simulink model "sim_orbit_min"  (Simulink 10.3)
settings: Solver=VariableStepAuto  StartTime=0.0  StopTime=.05*24*3600  FixedStep=1  MaxStep=1  RelTol=1e-3
InitFcn:
  | INIT_parametros;
  | dataAtm = data_atm('US1976');
undefined symbols (not defined in the file): A_transversal, a_world, b_world, Cbar, CI_angular, CI_lineal, e2_world, es2_world, GM, GRAV_MODEL, I, Jw, K, L, m, Omega0, Omega_max, P_peak, r_CG_in_G, SAT_SHAPE, Sbar, solar_cosep, solar_sinep, u_peak, WMM2025
libraries: aerolibgravity2 x1
settings Model: Creator=Allan  LastModifiedBy=RUSSO.MARTINEZ
settings SolverCC: AlgebraicLoopSolver=Auto
settings DataIOCC: SaveFormat=Dataset  SignalLoggingSaveFormat=Dataset
settings OptimizationCC: BlockReduction=off  ExpressionDepthLimit=128  LifeSpan=auto
settings DebuggingCC: SignalInfNanChecking=error  AlgebraicLoopMsg=none  UnderspecifiedInitializationDetection=Simplified  MergeDetectMultiDrivingBlocksExec=error  FcnCallInpInsideContextMsg=error  UnconnectedInputMsg=none  UnconnectedOutputMsg=none  UnconnectedLineMsg=none  StateNameClashWarn=none  SFUnexpectedBacktrackingDiag=error  SFNoUnconditionalDefaultTransitionDiag=error  SFExecutionAtInitializationDiag=warning  ArithmeticOperatorsInVariantConditions=error
settings HardwareCC: ProdBitPerPointer=64  ProdBitPerSizeT=64  ProdBitPerPtrDiffT=64  ProdLargestAtomicFloat=Float  ProdIntDivRoundTo=Zero  ProdEndianess=LittleEndian  ProdWordSize=64  ProdHWDeviceType=Intel->x86-64 (Windows64)
settings ModelReferenceCC: EnableRefExpFcnMdlSchedulingChecks=off  PropagateSignalLabelsOutOfModel=on
settings SFSimCC: SimUseLocalCustomCode=on  CustomCodeUndefinedFunction=FilterOut
settings RTWCC: RTWUseLocalCustomCode=on  GPUComputeCapability=5.0  DLArmComputeVersion=20.02.1
settings CodeAppCC: StateflowObjectComments=off
settings GRTTargetCC: TargetLangStandard=C99 (ISO)  CombineOutputUpdateFcns=on  GRTInterface=off
settings ConfigComp: CovMetricSettings=dwe  CovSaveCumulativeToWorkspaceVar=off  CovSaveSingleToWorkspaceVar=off  CovExternalEMLEnable=on  CovBoundaryAbsTol=1.0e-5

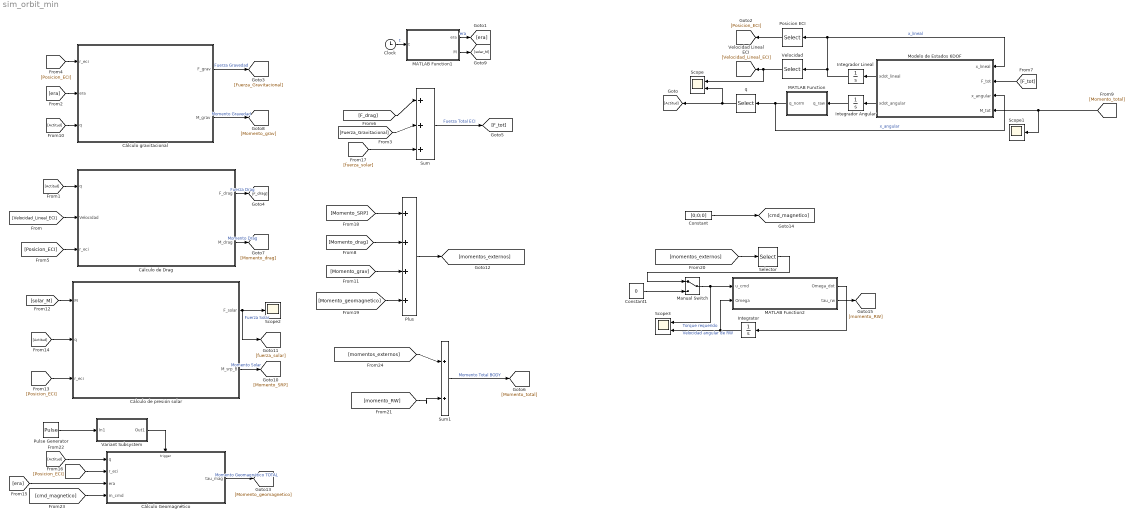
== system sim_orbit_min ==
  Clock : Clock
  Constant : Constant  Value=[0;0;0]  VectorParams1D=off
  Constant1 : Constant  Value=0
  Cálculo Geomagnético : Subsystem
  Cálculo de Drag : Subsystem
  Cálculo de presión solar : Subsystem
  Cálculo gravitacional : Subsystem
  Integrador Angular : Integrator  InitialCondition=CI_angular
  Integrador Lineal : Integrator  InitialCondition=CI_lineal
  Integrator : Integrator  InitialCondition=Omega0
  MATLAB Function : MATLAB Function  TreatAsAtomicUnit=on
  MATLAB Function1 : MATLAB Function  Priority=2  TreatAsAtomicUnit=on
  MATLAB Function2 : MATLAB Function  TreatAsAtomicUnit=on
  Manual Switch : ManualSwitch
  Modelo de Estados 6DOF : MATLAB Function  TreatAsAtomicUnit=on
  Plus : Sum  Inputs=++++
  Posicion ECI : Selector  InputPortWidth=6  IndexOptions=Index vector (dialog)  Indices=[1 2 3]  OutputSizes=1
  Pulse Generator : DiscretePulseGenerator  PulseType=Time based  Period=1  PulseWidth=50
  Scope : Scope  NumInputPorts=2
  Scope1 : Scope
  Scope2 : Scope
  Scope3 : Scope  NumInputPorts=2
  Selector : Selector  InputPortWidth=3  IndexOptions=Index vector (dialog)  Indices=[1]  OutputSizes=1
  Sum : Sum  Inputs=|+++
  Sum1 : Sum  Inputs=+|+
  Variant Subsystem : Subsystem  Variant=on
  "Velocidad " : Selector  InputPortWidth=6  IndexOptions=Index vector (dialog)  Indices=[4 5 6]  OutputSizes=1
  q : Selector  InputPortWidth=7  IndexOptions=Index vector (dialog)  Indices=[1 2 3 4]  OutputSizes=1
  wires:
  Clock/1 -> MATLAB Function1/1(t)  "t"
  Integrador Lineal/1 -> Posicion ECI/1, Modelo de Estados 6DOF/1(x_lineal), "Velocidad "/1  "x_lineal"
  "Velocidad "/1 -> Scope/1, [Velocidad_Lineal_ECI]
  Modelo de Estados 6DOF/1(xdot_lineal) -> Integrador Lineal/1
  Integrador Angular/1 -> MATLAB Function/1(q_raw)
  [Momento_total] -> Scope1/1, Modelo de Estados 6DOF/4(M_tot)
  [Actitud] -> Cálculo de Drag/1(q)
  [Velocidad_Lineal_ECI] -> Cálculo de Drag/2(Velocidad)
  MATLAB Function1/1(era) -> [era]  "era"
  Posicion ECI/1 -> [Posicion_ECI]
  [Posicion_ECI] -> Cálculo de Drag/3(r_eci)
  [era] -> Cálculo gravitacional/2(era)
  [Posicion_ECI] -> Cálculo gravitacional/1(r_eci)
  Cálculo gravitacional/1(F_grav) -> [Fuerza_Gravitacional]  "Fuerza Gravedad"
  [F_tot] -> Modelo de Estados 6DOF/2(F_tot)
  Modelo de Estados 6DOF/2(xdot_angular) -> Integrador Angular/1
  Cálculo de Drag/1(F_drag) -> [F_drag]  "Fuerza Drag"
  [F_drag] -> Sum/1
  Sum/1 -> [F_tot]  "Fuerza Total ECI"
  [Fuerza_Gravitacional] -> Sum/2
  Sum1/1 -> [Momento_total]  "Momento Total BODY"
  Cálculo de Drag/2(M_drag) -> [Momento_drag]  "Momento Drag"
  [Actitud] -> Cálculo gravitacional/3(q)
  Cálculo gravitacional/2(M_grav) -> [Momento_grav]  "Momento Gravedad"
  MATLAB Function1/2(M) -> [solar_M]
  [fuerza_solar] -> Sum/3
  [solar_M] -> Cálculo de presión solar/1(M)
  [Actitud] -> Cálculo de presión solar/2(q)
  [Posicion_ECI] -> Cálculo de presión solar/3(r_eci)
  Cálculo de presión solar/1(F_solar) -> [fuerza_solar], Scope2/1  "Fuerza Solar"
  Constant/1 -> [cmd_magnetico]
  [Actitud] -> Cálculo Geomagnético/1(q)
  [Posicion_ECI] -> Cálculo Geomagnético/2(r_eci)
  [era] -> Cálculo Geomagnético/3(era)
  [cmd_magnetico] -> Cálculo Geomagnético/4(m_cmd)
  Cálculo Geomagnético/1(tau_mag) -> [Momento_geomagnetico]  "Momento Geomagnético TOTAL"
  q/1 -> Scope/2, [Actitud]
  MATLAB Function/1(q_norm) -> Modelo de Estados 6DOF/3(x_angular), q/1  "x_angular"
  Cálculo de presión solar/2(M_srp_B) -> [Momento_SRP]  "Momento Solar"
  Pulse Generator/1 -> Variant Subsystem/1(In1)
  Variant Subsystem/1(Out1) -> Cálculo Geomagnético/Trigger
  [Momento_geomagnetico] -> Plus/4
  [Momento_grav] -> Plus/3
  [Momento_drag] -> Plus/2
  [Momento_SRP] -> Plus/1
  Plus/1 -> [momentos_externos]
  MATLAB Function2/1(Omega_dot) -> Integrator/1
  Integrator/1 -> MATLAB Function2/2(Omega), Scope3/2  "Velocidad angular de RW"
  [momentos_externos] -> Selector/1
  MATLAB Function2/2(tau_rw) -> [momento_RW]
  [momento_RW] -> Sum1/2
  [momentos_externos] -> Sum1/1
  Manual Switch/1 -> Scope3/1, MATLAB Function2/1(u_cmd)  "Torque requerido"
  Selector/1 -> Manual Switch/1
  Constant1/1 -> Manual Switch/2

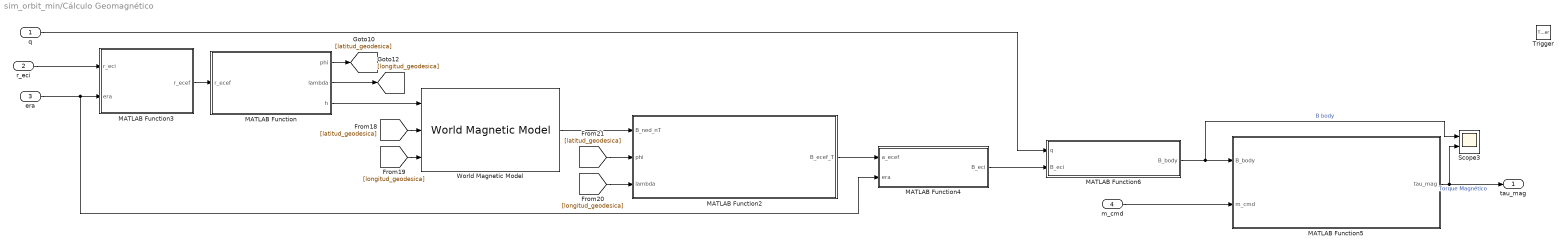
== system sim_orbit_min/Cálculo Geomagnético ==
  q : Inport
  r_eci : Inport  Port=2
  era : Inport  Port=3
  m_cmd : Inport  Port=4
  Trigger : TriggerPort  VariantControl=(inherit)  PortDimensions=1
  MATLAB Function : MATLAB Function  TreatAsAtomicUnit=on
  MATLAB Function2 : MATLAB Function  TreatAsAtomicUnit=on
  MATLAB Function3 : MATLAB Function  Priority=4  TreatAsAtomicUnit=on
  MATLAB Function4 : MATLAB Function  TreatAsAtomicUnit=on
  MATLAB Function5 : MATLAB Function  TreatAsAtomicUnit=on
  MATLAB Function6 : MATLAB Function  TreatAsAtomicUnit=on
  Scope3 : Scope  NumInputPorts=2
  World Magnetic Model : aerolibgravity2/World Magnetic Model  model=WMM2025 (2025-2030)  customFile='WMM2025.COF'  units=Metric (MKS)  time_in=off  month=January  day=1  year=2025  action=Error  h_out=off  dec_out=off  inc_out=off  ti_out=off
  tau_mag : Outport
  wires:
  [latitud_geodesica] -> MATLAB Function2/2(phi)
  [longitud_geodesica] -> World Magnetic Model/3
  MATLAB Function5/1(tau_mag) -> tau_mag/1, Scope3/2  "Torque Magnético"
  m_cmd/1 -> MATLAB Function5/2(m_cmd)
  MATLAB Function/1(phi) -> [latitud_geodesica]
  [latitud_geodesica] -> World Magnetic Model/2
  era/1 -> MATLAB Function4/2(era), MATLAB Function3/2(era)
  MATLAB Function6/1(B_body) -> Scope3/1, MATLAB Function5/1(B_body)  "B body"
  MATLAB Function/3(h) -> World Magnetic Model/1
  q/1 -> MATLAB Function6/1(q)
  [longitud_geodesica] -> MATLAB Function2/3(lambda)
  MATLAB Function/2(lambda) -> [longitud_geodesica]
  MATLAB Function4/1(B_eci) -> MATLAB Function6/2(B_eci)
  MATLAB Function2/1(B_ecef_T) -> MATLAB Function4/1(a_ecef)
  MATLAB Function3/1(r_ecef) -> MATLAB Function/1(r_ecef)
  World Magnetic Model/1 -> MATLAB Function2/1(B_ned_nT)
  r_eci/1 -> MATLAB Function3/1(r_eci)

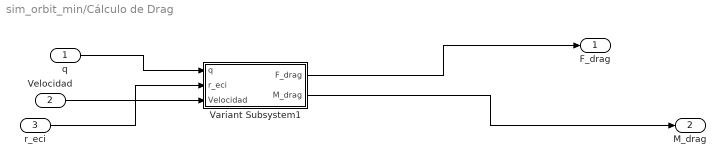
== system sim_orbit_min/Cálculo de Drag ==
  q : Inport
  Velocidad : Inport  Port=2
  r_eci : Inport  Port=3
  Variant Subsystem1 : Subsystem  Variant=on
  F_drag : Outport
  M_drag : Outport  Port=2  VectorParamsAs1DForOutWhenUnconnected=off
  wires:
  q/1 -> Variant Subsystem1/1(q)
  Velocidad/1 -> Variant Subsystem1/3(Velocidad)
  r_eci/1 -> Variant Subsystem1/2(r_eci)
  Variant Subsystem1/1(F_drag) -> F_drag/1
  Variant Subsystem1/2(M_drag) -> M_drag/1

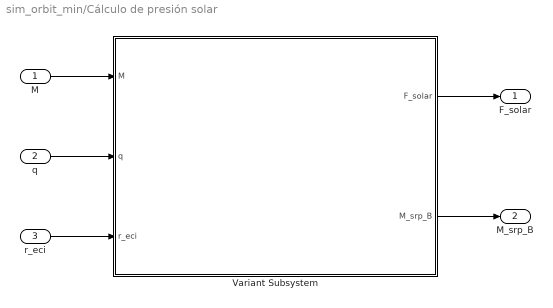
== system sim_orbit_min/Cálculo de presión solar ==
  M : Inport
  q : Inport  Port=2
  r_eci : Inport  Port=3
  Variant Subsystem : Subsystem  Variant=on
  F_solar : Outport
  M_srp_B : Outport  Port=2  VectorParamsAs1DForOutWhenUnconnected=off
  wires:
  M/1 -> Variant Subsystem/1(M)
  r_eci/1 -> Variant Subsystem/3(r_eci)
  q/1 -> Variant Subsystem/2(q)
  Variant Subsystem/1(F_solar) -> F_solar/1
  Variant Subsystem/2(M_srp_B) -> M_srp_B/1

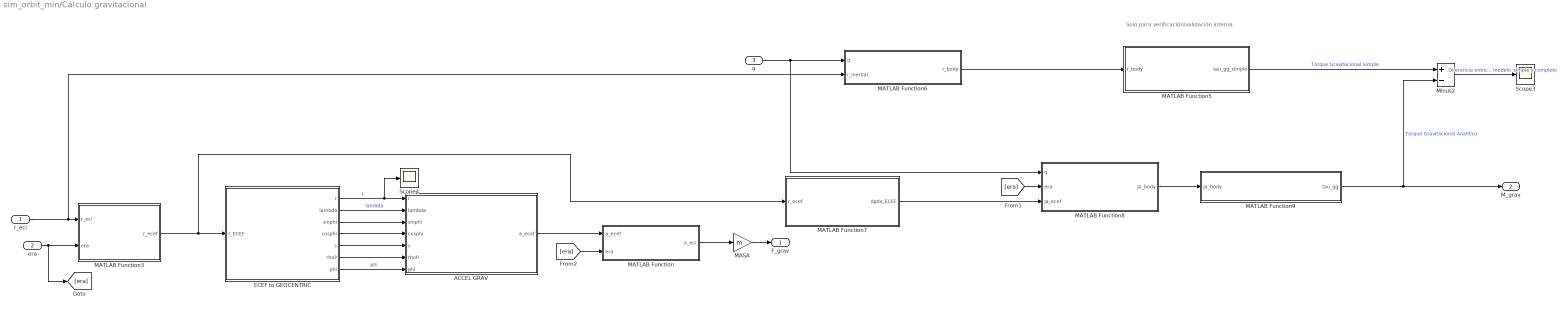
== system sim_orbit_min/Cálculo gravitacional ==
  note: Solo para verificación/validación interna.
  r_eci : Inport
  era : Inport  Port=2
  q : Inport  Port=3
  ACCEL GRAV : MATLAB Function  TreatAsAtomicUnit=on
  ECEF to GEOCENTRIC : MATLAB Function  TreatAsAtomicUnit=on
  MASA : Gain  Gain=m
  MATLAB Function : MATLAB Function  TreatAsAtomicUnit=on
  MATLAB Function3 : MATLAB Function  Priority=4  TreatAsAtomicUnit=on
  MATLAB Function5 : MATLAB Function  TreatAsAtomicUnit=on
  MATLAB Function6 : MATLAB Function  TreatAsAtomicUnit=on
  MATLAB Function7 : MATLAB Function  TreatAsAtomicUnit=on
  MATLAB Function8 : MATLAB Function  TreatAsAtomicUnit=on
  MATLAB Function9 : MATLAB Function  TreatAsAtomicUnit=on
  Minus2 : Sum  Inputs=+-
  Scope3 : Scope
  Scope4 : Scope
  F_grav : Outport  VectorParamsAs1DForOutWhenUnconnected=off
  M_grav : Outport  Port=2  VectorParamsAs1DForOutWhenUnconnected=off
  wires:
  MATLAB Function3/1(r_ecef) -> MATLAB Function7/1(r_ecef), ECEF to GEOCENTRIC/1(r_ECEF)
  ECEF to GEOCENTRIC/2(lambda) -> ACCEL GRAV/2(lambda)  "lambda"
  ECEF to GEOCENTRIC/1(r) -> Scope4/1, ACCEL GRAV/1(r)  "r"
  ECEF to GEOCENTRIC/3(sinphi) -> ACCEL GRAV/3(sinphi)
  ECEF to GEOCENTRIC/4(cosphi) -> ACCEL GRAV/4(cosphi)
  ECEF to GEOCENTRIC/5(s) -> ACCEL GRAV/5(s)
  ECEF to GEOCENTRIC/6(rhoP) -> ACCEL GRAV/6(rhoP)
  ACCEL GRAV/1(a_ecef) -> MATLAB Function/1(a_ecef)
  ECEF to GEOCENTRIC/7(phi) -> ACCEL GRAV/7(phi)  "phi"
  era/1 -> [era], MATLAB Function3/2(era)
  MASA/1 -> F_grav/1
  r_eci/1 -> MATLAB Function6/2(r_inertial), MATLAB Function3/1(r_eci)
  q/1 -> MATLAB Function8/1(q), MATLAB Function6/1(q)
  MATLAB Function/1(a_eci) -> MASA/1
  [era] -> MATLAB Function/2(era)
  MATLAB Function6/1(r_body) -> MATLAB Function5/1(r_body)
  MATLAB Function5/1(tau_gg_simple) -> Minus2/1  "Torque Gravitacional Simple"
  [era] -> MATLAB Function8/2(era)
  MATLAB Function7/1(dgdx_ECEF) -> MATLAB Function8/3(Ja_ecef)
  MATLAB Function8/1(Ja_body) -> MATLAB Function9/1(Ja_body)
  MATLAB Function9/1(tau_gg) -> Minus2/2, M_grav/1  "Torque Gravitacional Analítico"
  Minus2/1 -> Scope3/1  "Diferencia entre modelo  simple y completo"

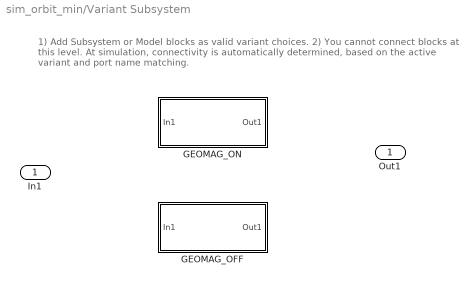
== system sim_orbit_min/Variant Subsystem ==
  note: 1) Add Subsystem or Model blocks as valid variant choices.
      | 2) You cannot connect blocks at this level. At simulation, connectivity is automatically
      | determined, based on the active variant and port name matching.
  In1 : Inport
  GEOMAG_OFF : Subsystem  VariantControl=GEOMAG_SEL == 2
  GEOMAG_ON : Subsystem  VariantControl=GEOMAG_SEL == 1
  Out1 : Outport

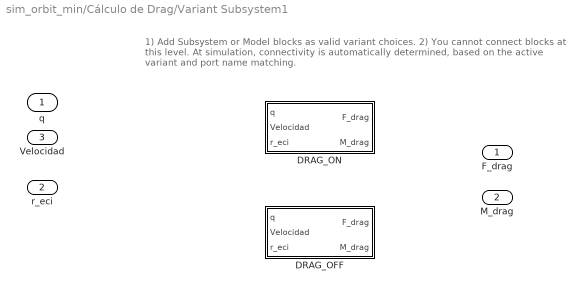
== system sim_orbit_min/Cálculo de Drag/Variant Subsystem1 ==
  note: 1) Add Subsystem or Model blocks as valid variant choices.
      | 2) You cannot connect blocks at this level. At simulation, connectivity is automatically
      | determined, based on the active variant and port name matching.
  q : Inport
  r_eci : Inport  Port=2
  Velocidad : Inport  Port=3
  DRAG_OFF : Subsystem  VariantControl=ATM_SEL == 3
  DRAG_ON : Subsystem  VariantControl=ATM_SEL < 3
  F_drag : Outport
  M_drag : Outport  Port=2

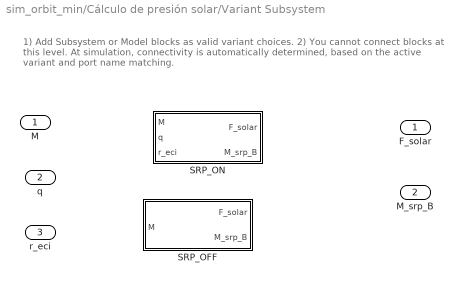
== system sim_orbit_min/Cálculo de presión solar/Variant Subsystem ==
  note: 1) Add Subsystem or Model blocks as valid variant choices.
      | 2) You cannot connect blocks at this level. At simulation, connectivity is automatically
      | determined, based on the active variant and port name matching.
  M : Inport
  q : Inport  Port=2
  r_eci : Inport  Port=3
  SRP_OFF : Subsystem  VariantControl=SRP_SEL == 2
  SRP_ON : Subsystem  VariantControl=SRP_SEL == 1
  F_solar : Outport
  M_srp_B : Outport  Port=2  VectorParamsAs1DForOutWhenUnconnected=off

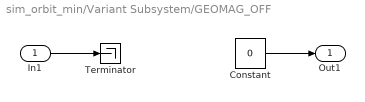
== system sim_orbit_min/Variant Subsystem/GEOMAG_OFF ==
  In1 : Inport
  Constant : Constant  Value=0
  Terminator : Terminator
  Out1 : Outport
  wires:
  In1/1 -> Terminator/1
  Constant/1 -> Out1/1

== system sim_orbit_min/Variant Subsystem/GEOMAG_ON ==
  In1 : Inport
  Out1 : Outport
  wires:
  In1/1 -> Out1/1

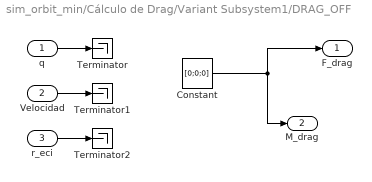
== system sim_orbit_min/Cálculo de Drag/Variant Subsystem1/DRAG_OFF ==
  q : Inport
  Velocidad : Inport  Port=2
  r_eci : Inport  Port=3
  Constant : Constant  Value=[0;0;0]
  Terminator : Terminator
  Terminator1 : Terminator
  Terminator2 : Terminator
  F_drag : Outport
  M_drag : Outport  Port=2  VectorParamsAs1DForOutWhenUnconnected=off
  wires:
  q/1 -> Terminator/1
  Velocidad/1 -> Terminator1/1
  r_eci/1 -> Terminator2/1
  Constant/1 -> M_drag/1, F_drag/1

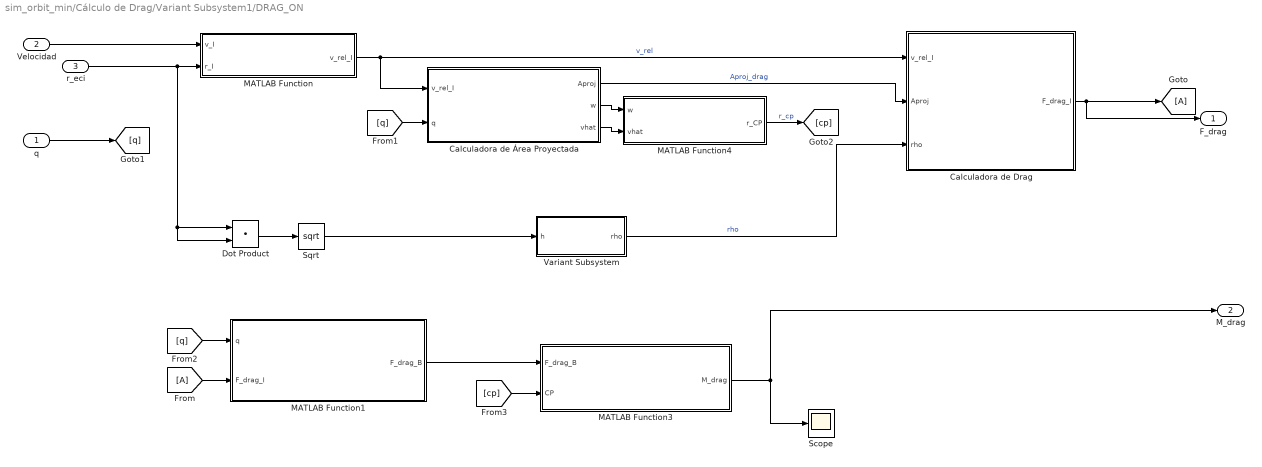
== system sim_orbit_min/Cálculo de Drag/Variant Subsystem1/DRAG_ON ==
  q : Inport
  Velocidad : Inport  Port=2
  r_eci : Inport  Port=3
  Calculadora de Drag : MATLAB Function  TreatAsAtomicUnit=on
  Calculadora de Área Proyectada : MATLAB Function  TreatAsAtomicUnit=on
  Dot Product : DotProduct  InputSameDT=on  OutDataTypeStr=Inherit: Inherit via internal rule
  MATLAB Function : MATLAB Function  TreatAsAtomicUnit=on
  MATLAB Function1 : MATLAB Function  TreatAsAtomicUnit=on
  MATLAB Function3 : MATLAB Function  TreatAsAtomicUnit=on
  MATLAB Function4 : MATLAB Function  TreatAsAtomicUnit=on
  Scope : Scope
  Sqrt : Sqrt  SaturateOnIntegerOverflow=on
  Variant Subsystem : Subsystem  Variant=on
  F_drag : Outport
  M_drag : Outport  Port=2
  wires:
  Variant Subsystem/1(rho) -> Calculadora de Drag/3(rho)  "rho"
  [A] -> MATLAB Function1/2(F_drag_I)
  Calculadora de Área Proyectada/1(Aproj) -> Calculadora de Drag/2(Aproj)  "Aproj_drag"
  Calculadora de Drag/1(F_drag_I) -> F_drag/1, [A]
  q/1 -> [q]
  MATLAB Function/1(v_rel_I) -> Calculadora de Drag/1(v_rel_I), Calculadora de Área Proyectada/1(v_rel_I)  "v_rel"
  r_eci/1 -> Dot Product/2, Dot Product/1, MATLAB Function/2(r_I)
  Calculadora de Área Proyectada/2(w) -> MATLAB Function4/1(w)
  MATLAB Function3/1(M_drag) -> M_drag/1, Scope/1
  Sqrt/1 -> Variant Subsystem/1(h)
  [q] -> MATLAB Function1/1(q)
  Calculadora de Área Proyectada/3(vhat) -> MATLAB Function4/2(vhat)
  MATLAB Function4/1(r_CP) -> [cp]  "r_cp"
  [cp] -> MATLAB Function3/2(CP)
  MATLAB Function1/1(F_drag_B) -> MATLAB Function3/1(F_drag_B)
  Velocidad/1 -> MATLAB Function/1(v_I)
  Dot Product/1 -> Sqrt/1
  [q] -> Calculadora de Área Proyectada/2(q)

== system sim_orbit_min/Cálculo de presión solar/Variant Subsystem/SRP_OFF ==
  M : Inport
  Constant : Constant  Value=0
  F_solar : Outport
  M_srp_B : Outport  Port=2  VectorParamsAs1DForOutWhenUnconnected=off
  wires:
  Constant/1 -> M_srp_B/1, F_solar/1

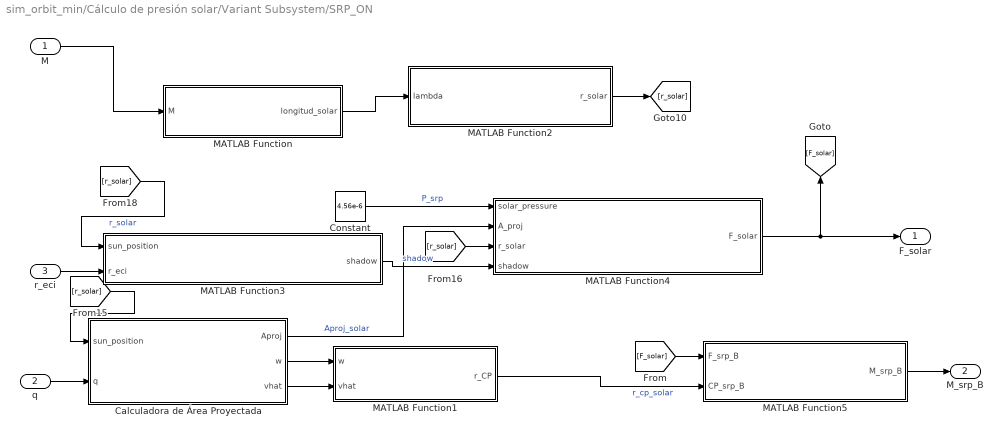
== system sim_orbit_min/Cálculo de presión solar/Variant Subsystem/SRP_ON ==
  M : Inport
  q : Inport  Port=2
  r_eci : Inport  Port=3
  Calculadora de Área Proyectada : MATLAB Function  TreatAsAtomicUnit=on
  Constant : Constant  Value=4.56e-6
  MATLAB Function : MATLAB Function  TreatAsAtomicUnit=on
  MATLAB Function1 : MATLAB Function  TreatAsAtomicUnit=on
  MATLAB Function2 : MATLAB Function  TreatAsAtomicUnit=on
  MATLAB Function3 : MATLAB Function  TreatAsAtomicUnit=on
  MATLAB Function4 : MATLAB Function  TreatAsAtomicUnit=on
  MATLAB Function5 : MATLAB Function  TreatAsAtomicUnit=on
  F_solar : Outport
  M_srp_B : Outport  Port=2  VectorParamsAs1DForOutWhenUnconnected=off
  wires:
  MATLAB Function/1(longitud_solar) -> MATLAB Function2/1(lambda)
  [r_solar] -> MATLAB Function3/1(sun_position)  "r_solar"
  MATLAB Function2/1(r_solar) -> [r_solar]
  Calculadora de Área Proyectada/3(vhat) -> MATLAB Function1/2(vhat)
  MATLAB Function4/1(F_solar) -> [F_solar], F_solar/1
  M/1 -> MATLAB Function/1(M)
  MATLAB Function3/1(shadow) -> MATLAB Function4/4(shadow)  "shadow"
  q/1 -> Calculadora de Área Proyectada/2(q)
  [r_solar] -> MATLAB Function4/3(r_solar)
  MATLAB Function1/1(r_CP) -> MATLAB Function5/2(CP_srp_B)  "r_cp_solar"
  r_eci/1 -> MATLAB Function3/2(r_eci)
  MATLAB Function5/1(M_srp_B) -> M_srp_B/1
  Calculadora de Área Proyectada/2(w) -> MATLAB Function1/1(w)
  [r_solar] -> Calculadora de Área Proyectada/1(sun_position)
  [F_solar] -> MATLAB Function5/1(F_srp_B)
  Calculadora de Área Proyectada/1(Aproj) -> MATLAB Function4/2(A_proj)  "Aproj_solar"
  Constant/1 -> MATLAB Function4/1(solar_pressure)  "P_srp"

== system sim_orbit_min/Cálculo de Drag/Variant Subsystem1/DRAG_ON/Variant Subsystem ==
  note: 1) Add Subsystem or Model blocks as valid variant choices.
      | 2) You cannot connect blocks at this level. At simulation, connectivity is automatically
      | determined, based on the active variant and port name matching.
  h : Inport
  ATM_EXP : Subsystem  VariantControl=ATM_SEL == 2
  ATM_US : Subsystem  VariantControl=ATM_SEL == 1
  rho : Outport

== system sim_orbit_min/Cálculo de Drag/Variant Subsystem1/DRAG_ON/Variant Subsystem/ATM_EXP ==
  h : Inport
  MATLAB Function2 : MATLAB Function  TreatAsAtomicUnit=on  VariantControl=Choice
  rho : Outport
  wires:
  h/1 -> MATLAB Function2/1(h)
  MATLAB Function2/1(rho) -> rho/1  "Densidad exponencial"

== system sim_orbit_min/Cálculo de Drag/Variant Subsystem1/DRAG_ON/Variant Subsystem/ATM_US ==
  h : Inport
  MATLAB Function5 : MATLAB Function  TreatAsAtomicUnit=on  VariantControl=Choice_1
  rho : Outport
  wires:
  h/1 -> MATLAB Function5/1(h)
  MATLAB Function5/1(rho) -> rho/1  "Densidad US 1962"

== matlab function MATLAB Function1 ==
  data: t input double; era output double; M output double; jd_ut_inicial parameter double
function [era,M] = MD_era(t,jd_ut_inicial)
[era,M] = MD_era(t,jd_ut_inicial);
end

== matlab function Cálculo de Drag/Variant Subsystem1/DRAG_ON/MATLAB Function ==
  data: v_I input double; r_I input double; v_rel_I output double
function v_rel_I = MD_velocidad_relativa(v_I,r_I)
v_rel_I = MD_velocidad_relativa(v_I,r_I);
end

== matlab function Cálculo gravitacional/ACCEL GRAV ==
  data: r input double; lambda input double; sinphi input double; cosphi input double; s input double; rhoP input double; a_ecef output double; Cbar parameter double; Sbar parameter double; K parameter double; GM parameter double; phi input double
function a_ecef = MD_aceleracion_geopotencial(r, lambda, sinphi, cosphi, s, rhoP, Cbar, Sbar, K, GM, phi)
     a_ecef = MD_aceleracion_geopotencial(r, lambda, sinphi, cosphi, s, rhoP, Cbar, Sbar, K, GM, phi);
end

== matlab function Cálculo gravitacional/MATLAB Function3 ==
  data: r_eci input double; r_ecef output double; era input double; C_FIX_val parameter double
function r_ecef = MT_ECI2ECEF(r_eci, era,C_FIX_val)
 r_ecef = MT_ECI2ECEF(r_eci, era, C_FIX_val);
end

== matlab function Modelo de Estados 6DOF ==
  data: x_lineal input double; xdot_lineal output double; F_tot input double; x_angular input double; M_tot input double; xdot_angular output double; m parameter double; I parameter double
%% Modelo de estados para un cuerpo rigido con x_lineal = [r(3x1);v(3x1)] y a_angular = [q(4x1);omega(3x1)]
function [xdot_lineal, xdot_angular] = MD_modelo_de_estados(x_lineal,F_tot,x_angular,M_tot,m, I)
    [xdot_lineal, xdot_angular] = MD_modelo_de_estados(x_lineal,F_tot,x_angular,M_tot,m,I);
end

== matlab function Cálculo gravitacional/ECEF to GEOCENTRIC ==
  data: r output double; r_ECEF input double; lambda output double; sinphi output double; cosphi output double; s output double; rhoP output double; phi output double
function [r, lambda, sinphi, cosphi, s, rhoP,phi] = MT_ECEF2GEOCENTRIC(r_ECEF)
    [r, lambda, sinphi, cosphi, s, rhoP,phi] = MT_ECEF2GEOCENTRIC(r_ECEF);
end

== matlab function Cálculo gravitacional/MATLAB Function5 ==
  data: r_body input double; tau_gg_simple output double; GM parameter double; I parameter double
function tau_gg_simple = MD_torque_grav_simple(r_body, GM, I)
 tau_gg_simple = MD_torque_grav_simple(r_body, I,GM);
end

== matlab function Cálculo gravitacional/MATLAB Function7 ==
  data: r_ecef input double; dgdx_ECEF output double; a_world parameter double; Cbar parameter double; Sbar parameter double; K parameter double; GM parameter double; GRAV_MODEL parameter double
function dgdx_ECEF = MD_Ja_analitico(r_ecef, a_world, Cbar, Sbar, K, GM, GRAV_MODEL)
         dgdx_ECEF = MD_Ja_analitico(r_ecef, a_world, Cbar, Sbar, K, GM, GRAV_MODEL);
end

== matlab function Cálculo de Drag/Variant Subsystem1/DRAG_ON/Calculadora de Drag ==
  data: v_rel_I input double; Aproj input double; rho input double; F_drag_I output double; CD parameter double
function F_drag_I = MD_drag(v_rel_I, Aproj, rho, CD)
 F_drag_I = MD_drag(v_rel_I,Aproj, rho,CD);
end

== matlab function Cálculo de Drag/Variant Subsystem1/DRAG_ON/Calculadora de Área Proyectada ==
  data: v_rel_I input double; q input double; Aproj output double; A_transversal parameter double; w output double; vhat output double; SAT_SHAPE parameter double
function [Aproj,w,vhat] = MT_area_proyectada(v_rel_I, q, A_transversal, SAT_SHAPE)
         [Aproj,w,vhat] = MT_area_proyectada(v_rel_I, q, A_transversal, SAT_SHAPE);
end

== matlab function Cálculo gravitacional/MATLAB Function ==
  data: a_eci output double; a_ecef input double; era input double; C_FIX_val parameter double
function a_eci = MT_ECEF2ECI(a_ecef, era,C_FIX_val)
    a_eci = MT_ECEF2ECI(a_ecef, era,C_FIX_val);
end

== matlab function Cálculo de Drag/Variant Subsystem1/DRAG_ON/MATLAB Function1 ==
  data: q input double; F_drag_B output double; F_drag_I input double
function  F_drag_B= MT_ECI2BODY(q,F_drag_I)
  F_drag_B= MT_ECI2BODY(q,F_drag_I);
end

== matlab function Cálculo de Drag/Variant Subsystem1/DRAG_ON/MATLAB Function3 ==
  data: F_drag_B input double; M_drag output double; CP input double; l_minimo_drag parameter double
function M_drag = MD_momento_drag(F_drag_B, CP,l_minimo_drag)
 M_drag = MD_momento_drag(F_drag_B, CP,l_minimo_drag);
end

== matlab function MATLAB Function2 ==
  data: u_cmd input double; Omega_dot output double; Omega input double; tau_rw output double; Jw parameter double; u_peak parameter double; Omega_max parameter double; P_peak parameter double
function [Omega_dot, tau_rw] = MD_RW(u_cmd, Omega, Jw, u_peak, Omega_max, P_peak)
 [Omega_dot, tau_rw] = MD_RW(u_cmd, Omega, Jw, u_peak, Omega_max, P_peak);

== matlab function Cálculo gravitacional/MATLAB Function6 ==
  data: q input double; r_body output double; r_inertial input double
function  r_body= MT_ECI2BODY(q,r_inertial)
  r_body= MT_ECI2BODY(q,r_inertial);
end

== matlab function Cálculo Geomagnético/MATLAB Function3 ==
  data: r_eci input double; r_ecef output double; era input double; C_FIX_val parameter double
function r_ecef = MT_ECI2ECEF(r_eci, era,C_FIX_val)
 r_ecef = MT_ECI2ECEF(r_eci, era,C_FIX_val);
end

== matlab function Cálculo Geomagnético/MATLAB Function ==
  data: r_ecef input double; phi output double; lambda output double; h output double; a_world parameter double; b_world parameter double; e2_world parameter double; es2_world parameter double
function [phi, lambda, h] = MT_ECEF2GEODETIC(r_ecef,a_world, b_world, e2_world, es2_world)
 [phi, lambda, h] = MT_ECEF2GEODETIC(r_ecef,a_world,b_world,e2_world,es2_world);

== matlab function Cálculo Geomagnético/MATLAB Function2 ==
  data: B_ned_nT input double; phi input double; B_ecef_T output double; lambda input double
function B_ecef_T = MT_NED2ECEF(B_ned_nT, phi, lambda)
 B_ecef_T = MT_NED2ECEF(B_ned_nT, phi, lambda);

== matlab function Cálculo Geomagnético/MATLAB Function4 ==
  data: B_eci output double; a_ecef input double; era input double; C_FIX_val parameter double
function B_eci = MT_ECEF2ECI(a_ecef, era,C_FIX_val)
    B_eci = MT_ECEF2ECI(a_ecef, era,C_FIX_val);
end

== matlab function Cálculo Geomagnético/MATLAB Function6 ==
  data: q input double; B_body output double; B_eci input double
function  B_body= MT_ECI2BODY(q,B_eci)
  B_body= MT_ECI2BODY(q,B_eci);
end

== matlab function Cálculo Geomagnético/MATLAB Function5 ==
  data: B_body input double; m_res parameter double; tau_mag output double; m_cmd input double
function tau_mag = MD_torque_magnetico(B_body, m_res, m_cmd)
 tau_mag = MD_torque_magnetico(B_body, m_res, m_cmd);

== matlab function MATLAB Function ==
  data: q_raw input double; q_norm output double
function q_norm = MD_normalize_q(q_raw)
 q_norm = MD_normalize_q(q_raw);
end

== matlab function Cálculo de Drag/Variant Subsystem1/DRAG_ON/MATLAB Function4 ==
  data: w input double; vhat input double; r_CP output double; L parameter double; r_CG_in_G parameter double
function r_CP = MD_cp_calculator(w, vhat, L, r_CG_in_G)
r_CP = MD_cp_calculator(w, vhat, L,r_CG_in_G);
end

== matlab function Cálculo gravitacional/MATLAB Function8 ==
  data: q input double; era input double; Ja_body output double; Ja_ecef input double; C_FIX_val parameter double
function Ja_body = MT_ECEF2BODY_matrix(q,era,Ja_ecef,C_FIX_val)
Ja_body = MT_ECEF2BODY_matrix(q,era,Ja_ecef,C_FIX_val);
end

== matlab function Cálculo de Drag/Variant Subsystem1/DRAG_ON/Variant Subsystem/ATM_EXP/MATLAB Function2 ==
  data: h input double; rho output double
function rho = MD_densidad(h)
rho = MD_densidad(h);
end

== matlab function Cálculo de Drag/Variant Subsystem1/DRAG_ON/Variant Subsystem/ATM_US/MATLAB Function5 ==
  data: h input double; rho output double; dataAtm parameter double
function rho = c_atmUS1962(h,dataAtm) 
 rho = c_atmUS1962(h,dataAtm);

== matlab function Cálculo gravitacional/MATLAB Function9 ==
  data: Ja_body input double; tau_gg output double; I parameter double
function tau_gg = MD_momento_gravitatorio(Ja_body,I)
tau_gg = MD_momento_gravitatorio(Ja_body,I);
end

== matlab function Cálculo de presión solar/Variant Subsystem/SRP_ON/Calculadora de Área Proyectada ==
  data: sun_position input double; q input double; Aproj output double; A_transversal parameter double; w output double; vhat output double; SAT_SHAPE parameter double
function [Aproj,w,vhat] = MT_area_proyectada(sun_position, q, A_transversal, SAT_SHAPE)
[Aproj,w,vhat] = MT_area_proyectada(sun_position, q, A_transversal, SAT_SHAPE);
end

== matlab function Cálculo de presión solar/Variant Subsystem/SRP_ON/MATLAB Function ==
  data: M input double; longitud_solar output double; solar_omegas parameter double
function longitud_solar = MD_sun_position(M,solar_omegas)
longitud_solar = MD_sun_position(M,solar_omegas);
end

== matlab function Cálculo de presión solar/Variant Subsystem/SRP_ON/MATLAB Function1 ==
  data: w input double; vhat input double; r_CP output double; L parameter double; r_CG_in_G parameter double
function r_CP = MD_cp_calculator(w, vhat, L, r_CG_in_G)
 r_CP = MD_cp_calculator(w, vhat, L,r_CG_in_G);
end

== matlab function Cálculo de presión solar/Variant Subsystem/SRP_ON/MATLAB Function2 ==
  data: lambda input double; r_solar output double; solar_cosep parameter double; solar_sinep parameter double
function r_solar = MT_SOLAR_GEOCENTRIC2ECI(lambda, solar_cosep, solar_sinep)
 r_solar = MT_SOLAR_GEOCENTRIC2ECI(lambda,solar_cosep,solar_sinep);
end

== matlab function Cálculo de presión solar/Variant Subsystem/SRP_ON/MATLAB Function3 ==
  data: sun_position input double; shadow output double; r_eci input double
function shadow = MD_shadow_function(sun_position,r_eci)
 shadow = MD_shadow_function(sun_position,r_eci);
end

== matlab function Cálculo de presión solar/Variant Subsystem/SRP_ON/MATLAB Function4 ==
  data: solar_pressure input double; F_solar output double; A_proj input double; r_solar input double; Cr parameter double; shadow input double
function F_solar = MD_solar_force(solar_pressure,A_proj,r_solar, Cr,shadow)
 F_solar = MD_solar_force(solar_pressure,A_proj,Cr,r_solar,shadow);

== matlab function Cálculo de presión solar/Variant Subsystem/SRP_ON/MATLAB Function5 ==
  data: F_srp_B input double; M_srp_B output double; CP_srp_B input double
function M_srp_B = MD_momento_srp(F_srp_B, CP_srp_B)
 M_srp_B = MD_momento_srp(F_srp_B, CP_srp_B);
